simulink model "Viertel_Fahrzeug_model"  (R2023b)
settings: Solver=VariableStepAuto  StartTime=0.0  StopTime=10.0  RelTol=1e-3
settings Model: Creator=Balaji  LastModifiedBy=Balaji

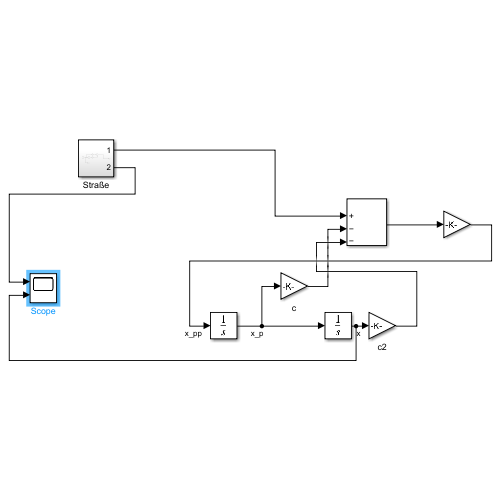
[thumbnail: Simulink's stored preview of the top-level diagram]
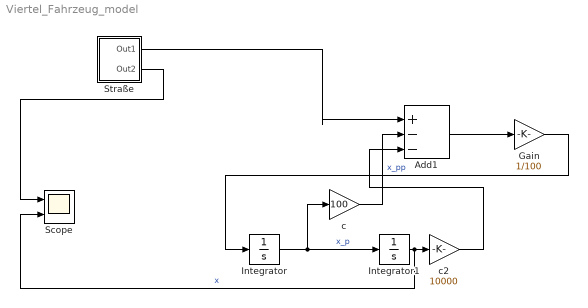
== system Viertel_Fahrzeug_model ==
  Add1 : Sum  Inputs=|+--
  Gain : Gain  Gain=1/100
  Integrator : Integrator
  Integrator1 : Integrator
  Scope : Scope  NumInputPorts=2
  Straße : Subsystem
  c : Gain  Gain=100
  c2 : Gain  Gain=10000
  wires:
  Gain/1 -> Integrator/1  "x_pp"
  Integrator/1 -> c/1, Integrator1/1  "x_p"
  c/1 -> Add1/2
  Integrator1/1 -> Scope/2, c2/1  "x"
  c2/1 -> Add1/3
  Add1/1 -> Gain/1
  Straße/1(Out1) -> Add1/1
  Straße/2(Out2) -> Scope/1

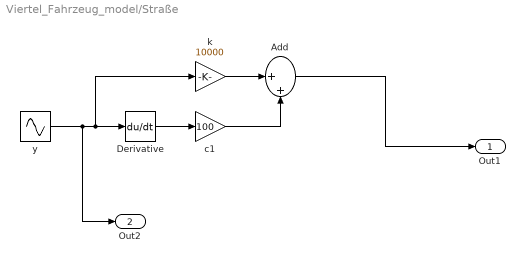
== system Viertel_Fahrzeug_model/Straße ==
  Add : Sum  Inputs=|++
  Derivative : Derivative
  c1 : Gain  Gain=100
  k : Gain  Gain=10000
  y : Sin  Amplitude=0.1  Frequency=0.5  SampleTime=0
  Out1 : Outport
  Out2 : Outport  Port=2
  wires:
  Add/1 -> Out1/1
  y/1 -> Out2/1, k/1, Derivative/1
  k/1 -> Add/1
  c1/1 -> Add/2
  Derivative/1 -> c1/1
